simulink library "IOBlock_Library_TTC580"  (R2021a)
settings: Solver=ode45  StartTime=0.0  StopTime=10.0  RelTol=1e-3
PreLoadFcn:
  | addpath(genpath(fileparts(which('IOBlock_Library_TTC580'))));
  | %addpath(genpath(fileparts(which('IOBlock_Library_TTC580.mdl'))))
  | try
  | addpath(genpath([fileparts(which('IOBlock_Library_TTC580')),'\..\DBC_Importer']));
  | addpath(genpath([fileparts(which('IOBlock_Library_TTC580')),'\..\EEPROM_Importer']));
  | addpath(genpath([fileparts(which('IOBlock_Library_TTC580')),'\..\UserDoc']));
  | catch
  | warning('IOBlock_Library_TTC580: add path to DBC_Importer and EEPROM_Importer manually');
  | end
  | try
  | if exist('..\CustomPackage\scripts\OpenAllPackages.m','file')
  |      run('..\CustomPackage\scripts\OpenAllPackages.m'); %always available, ggf. empty
  | end
  | catch
  | warning('A problem occurred opening automatically the CustomPackage. Please open libraries manually');
  | end
  | try
  | set_param(0,'EditorSmartEditingHotParam','off');
  | catch
  | warning('Simlink preferences for ''Edit key parameter when adding new blocks'' needs to be unchecked manually');
  | end
undefined symbols (not defined in the file or in its folder): ADC_Absolute_10V, ADC_Absolute_32V, ADC_Absolute_5V, ADC_BoardTemp, ADC_ChannelInit, ADC_Current, ADC_Get, ADC_K15_, ADC_Ratiometric_10V, ADC_Ratiometric_5V, ADC_Resistive, ADC_SensorSupply, ADC_UBAT, bit_packing, bit_unpacking, CAN_ConfigMsg, compare2error, compare2FET_PROT_REENABLE, crc32_calc_intern, CRC32_EEPROM_Read, CRC32_EEPROM_Write, DIAG_EnterSafestate, DIAG_Status, DIAG_Status_internal, EEPROM_Mirror, EEPROM_Read, EEPROM_Read_OffsetIn, EEPROM_Read_Raw, EEPROM_Write, EEPROM_Write_OffsetIn, EEPROM_Write_Raw, EnterSafestate, FPU_Handler, Get_DI, Get_DI_VarThreshold, Get_K15_, Get_Pulse_Freq_Curr, Get_Pulse_Freq_Volt, Get_WakeUp, GetDateAndTime, IO_ADC_ResetProtection, IO_Blk_Lib_TTC500, IO_CAN_ReadMsg, IO_CAN_WriteMsg, IO_DI_Get, IO_DI_Init, IO_DI_Init_Var, IO_DO_GetCur, IO_DO_GetVoltage, IO_DO_Init, IO_DO_ResetProtection, IO_DO_Set, IO_Driver_GetSerialNumber, IO_Driver_GetVersionOfDriver, IO_Driver_GetVersionOfFPGA, IO_EEPROM_GetStatus, IO_EEPROM_Init, IO_EEPROM_Read_raw, IO_EEPROM_Write, IO_EEPROM_Write_OffsetIn ... (+73)
libraries: simulink x43
(part 2 of 18)

== system IOBlock_Library_TTC580/CAN  Blocks TTC580 IOlib ==
  OR_TX : S-Function  FunctionName=sfix_bitop  Parameters=UseBitMask,NumInputPorts,BitMask,BitMaskRealWorld,logicop  SFunctionDeploymentMode=off  EnableBusSupport=off  mask(Bitwise Operator){logicop=OR, UseBitMask=off, NumInputPorts=2, BitMask=bin2dec('11011001'), BitMaskRealWorld=Stored Integer}
      mask prompts: logicop "Operator:"; UseBitMask "Use bit mask ..."; NumInputPorts "Number of input ports:"; BitMask "Bit Mask"; BitMaskRealWorld "Treat mask as:"
      mask help:
      | Perform the specified bitwise operation on the inputs. The output data type should represent zero exactly.
      | CAN buffer-outputs of the bit_packing blocks may be merged to a single CAN buffer (uint32[2]) which may be sent out by CAN_Write blocks.
      mask init:
      | if UseBitMask
      |   [m,n] = size(BitMask);
      |   if ischar(BitMask)
      |     len = m;
      |     n = 1;
      |   else
      |     len = m * n;
      |   end
      |   internalBitMask = zeros(m,n);
      |   if isnumeric(BitMask)
      |     for i=1:len,
      |       internalBitMask(i) = BitMask(i);
      |     end
      |   elseif ischar(BitMask)
      |     for i=1:m,
      |       internalBitMask(i) = hex2dec(BitMask(i,:));
      |     end
      |   elseif iscell(BitMask)
      |     for i=1:len,
      |       if isnumeric( BitMask{i} )
      |         internalBitMask(i) = BitMask{i};
      |       elseif ischar( BitMask{i} )
      |         internalBitMask(i) = hex2dec(BitMask{i});
      |       else
      |         errordlg(['Data type is not supported at cell item ', num2str(i) ]);
      |       end
      |     end
      |   end
      |   BitMask = internalBitMask;
      |   if len == 1
      |      if BitMaskRealWorld == 1 || BitMask(1) < 0
      |        str=num2str(BitMask(1));
      |      else
      |        str=['0x',dec2hex(floor(BitMask(1)))];
      |      end
      |   else
      |      str='Masks';
      |   end
      | else
      |   BitMask = 0;
      |   str='';
      | end
      mask TypeOptions logicop: AND | OR | NAND | NOR | XOR | NOT
      mask Callback logicop: fixptdialog(gcbh)
      mask Callback UseBitMask: fixptdialog(gcbh)
      mask TypeOptions BitMaskRealWorld: Real World Value | Stored Integer
      mask Display: fprintf(['Bitwise\n',logicop,'\n',str])
  ReadMsg_CAN : Subsystem  LoadFcn=|  mask(ReadMsg_CAN_Code){SampleTime=-1, ttlib=IO_Blk_Lib_TTC500, ttDescription=ReadMsg_CAN, tt_iolib_version=0.26, channel=IO_CAN_CHANNEL_0, mode=IO_CAN_MSG_READ, id_format=IO_CAN_STD_FRAME, id=hex2dec('123')}
      | try
      | %
      | %Upgrade Information - standard BEGIN
      | new_color = 'blue';
      | new_ver = '0.26';
      | act_ver = get_param(gcb,'tt_iolib_version');
      | if not(strcmp(act_ver,new_ver))
      |     disp(['Upgrade block: ',gcb,char(10),'       Version: ',act_ver,' to ',new_ver]);
      |     %switch - case for specific upgrade information e.g. additional parameter required 
      |     %Change appearance and version information
      |     set_param(gcb,'ForegroundColor',new_color);
      |     set_param(gcb,'tt_iolib_version',new_ver);
      | end
      | %Upgrade Information - standard END
      | catch
      | %Standard catch section BEGIN
      | errordlg('An error occurred in a callback of the TTC580-BlockLib. Please open the Diagnostic Viewer for further details');
      | disp(' ');
      | disp('------------------------------------------------------------');
      | disp('An error occurred in a callback of the TTC580-BlockLib.');
      | disp(['Please check the parameters in the mask of ',gcb]);
      | disp('If you do not encounter any violations, then please '); 
      | disp('copy the following lines and report this to support@ttcontrol.com ');
      | disp('<< begin of error message dump >>');
      | disp(['Version of TTC580-BlockLib: ', get_param(gcb,'tt_iolib_version')]);
      | disp(get_param(gcb,'ttDescription'));
      | disp(gcb);
      | x=lasterror;disp(x.message);
      | disp(get_param(gcb,'MaskValues'));
      | disp(version);
      | disp(computer);
      | disp('<< end of error message dump >>');
      | disp('------------------------------------------------------------');
      | disp(' ');
      | %Standard catch section END
      | end
      mask help: Reads a message from a given message object.
      mask init: same as IOBlock_Library_TTC580/ADC Blocks TTC580 IOlib/ADC_Absolute_10V
      settings: CopyFcn=%deleted
      mask Help: web([which('usermanual.html'),'#',lower(get_param(gcb,'ttDescription'))])
      mask TypeOptions channel: IO_CAN_CHANNEL_0  | IO_CAN_CHANNEL_1 | IO_CAN_CHANNEL_2 | IO_CAN_CHANNEL_3 | IO_CAN_CHANNEL_4 | IO_CAN_CHANNEL_5 | IO_CAN_CHANNEL_6
      mask Callback channel: %
      mask Callback mode: %
      mask TypeOptions id_format: IO_CAN_STD_FRAME | IO_CAN_EXT_FRAME
      mask Callback id_format: %
      mask Callback id: %
  ReadMsg_CAN_derated : Subsystem  LoadFcn=|  mask(ReadMsg_CAN_derated_Code){SampleTime=-1, ttlib=IO_Blk_Lib_TTC500, ttDescription=ReadMsg_CAN_derated, tt_iolib_version=0.26, channel=IO_CAN_CHANNEL_0, mode=IO_CAN_MSG_READ, id_format=IO_CAN_STD_FRAME, id=hex2dec('123'), derate=10}
      | try
      | %
      | %Upgrade Information - standard BEGIN
      | new_color = 'blue';
      | new_ver = '0.26';
      | act_ver = get_param(gcb,'tt_iolib_version');
      | if not(strcmp(act_ver,new_ver))
      |     disp(['Upgrade block: ',gcb,char(10),'       Version: ',act_ver,' to ',new_ver]);
      |     %switch - case for specific upgrade information e.g. additional parameter required 
      |     %Change appearance and version information
      |     set_param(gcb,'ForegroundColor',new_color);
      |     set_param(gcb,'tt_iolib_version',new_ver);
      | end
      | %Upgrade Information - standard END
      | catch
      | %Standard catch section BEGIN
      | errordlg('An error occurred in a callback of the TTC580-BlockLib. Please open the Diagnostic Viewer for further details');
      | disp(' ');
      | disp('------------------------------------------------------------');
      | disp('An error occurred in a callback of the TTC580-BlockLib.');
      | disp(['Please check the parameters in the mask of ',gcb]);
      | disp('If you do not encounter any violations, then please '); 
      | disp('copy the following lines and report this to support@ttcontrol.com ');
      | disp('<< begin of error message dump >>');
      | disp(['Version of TTC580-BlockLib: ', get_param(gcb,'tt_iolib_version')]);
      | disp(get_param(gcb,'ttDescription'));
      | disp(gcb);
      | x=lasterror;disp(x.message);
      | disp(get_param(gcb,'MaskValues'));
      | disp(version);
      | disp(computer);
      | disp('<< end of error message dump >>');
      | disp('------------------------------------------------------------');
      | disp(' ');
      | %Standard catch section END
      | end
      mask help:
      | Representation of the ReadMsg_CAN function call, with derate
      | functionality.
      mask init: same as IOBlock_Library_TTC580/ADC Blocks TTC580 IOlib/ADC_Absolute_10V
      settings: CopyFcn=%deleted
      mask Help: web([which('usermanual.html'),'#',lower(get_param(gcb,'ttDescription'))])
      mask TypeOptions channel: IO_CAN_CHANNEL_0  | IO_CAN_CHANNEL_1 | IO_CAN_CHANNEL_2 | IO_CAN_CHANNEL_3 | IO_CAN_CHANNEL_4 | IO_CAN_CHANNEL_5 | IO_CAN_CHANNEL_6
      mask Callback channel: %
      mask Callback mode: %
      mask TypeOptions id_format: IO_CAN_STD_FRAME | IO_CAN_EXT_FRAME
      mask Callback id_format: %
      mask Callback id: %
      mask Callback derate: %
  WriteMsg_CAN : Subsystem  LoadFcn=|  mask(WriteMsg_CAN_Code){SampleTime=-1, ttlib=IO_Blk_Lib_TTC500, ttDescription=WriteMsg_CAN, tt_iolib_version=0.26, channel=IO_CAN_CHANNEL_0, mode=IO_CAN_MSG_WRITE, id_format=IO_CAN_STD_FRAME, id=hex2dec('123'), length=8}
      | try
      | %
      | %Upgrade Information - standard BEGIN
      | new_color = 'blue';
      | new_ver = '0.26';
      | act_ver = get_param(gcb,'tt_iolib_version');
      | if not(strcmp(act_ver,new_ver))
      |     disp(['Upgrade block: ',gcb,char(10),'       Version: ',act_ver,' to ',new_ver]);
      |     %switch - case for specific upgrade information e.g. additional parameter required 
      |     %Change appearance and version information
      |     set_param(gcb,'ForegroundColor',new_color);
      |     set_param(gcb,'tt_iolib_version',new_ver);
      | end
      | %Upgrade Information - standard END
      | catch
      | %Standard catch section BEGIN
      | errordlg('An error occurred in a callback of the TTC580-BlockLib. Please open the Diagnostic Viewer for further details');
      | disp(' ');
      | disp('------------------------------------------------------------');
      | disp('An error occurred in a callback of the TTC580-BlockLib.');
      | disp(['Please check the parameters in the mask of ',gcb]);
      | disp('If you do not encounter any violations, then please '); 
      | disp('copy the following lines and report this to support@ttcontrol.com ');
      | disp('<< begin of error message dump >>');
      | disp(['Version of TTC580-BlockLib: ', get_param(gcb,'tt_iolib_version')]);
      | disp(get_param(gcb,'ttDescription'));
      | disp(gcb);
      | x=lasterror;disp(x.message);
      | disp(get_param(gcb,'MaskValues'));
      | disp(version);
      | disp(computer);
      | disp('<< end of error message dump >>');
      | disp('------------------------------------------------------------');
      | disp(' ');
      | %Standard catch section END
      | end
      mask help: Transmits a CAN message, using the given channel and message object.
      mask init: same as IOBlock_Library_TTC580/ADC Blocks TTC580 IOlib/ADC_Absolute_10V
      settings: CopyFcn=%deleted
      mask Help: web([which('usermanual.html'),'#',lower(get_param(gcb,'ttDescription'))])
      mask TypeOptions channel: IO_CAN_CHANNEL_0  | IO_CAN_CHANNEL_1 | IO_CAN_CHANNEL_2 | IO_CAN_CHANNEL_3 | IO_CAN_CHANNEL_4 | IO_CAN_CHANNEL_5 | IO_CAN_CHANNEL_6
      mask Callback channel: %
      mask Callback mode: %
      mask TypeOptions id_format: IO_CAN_STD_FRAME | IO_CAN_EXT_FRAME
      mask Callback id_format: %
      mask Callback id: %
      mask Callback length: %
  WriteMsg_CAN_derated : Subsystem  LoadFcn=|  mask(WriteMsg_CAN_derated_Code){SampleTime=-1, ttlib=IO_Blk_Lib_TTC500, ttDescription=WriteMsg_CAN_derated, tt_iolib_version=0.26, channel=IO_CAN_CHANNEL_0, mode=IO_CAN_MSG_WRITE, id_format=IO_CAN_STD_FRAME, id=hex2dec('123'), length=8, derate=10}
      | try
      | %
      | %Upgrade Information - standard BEGIN
      | new_color = 'blue';
      | new_ver = '0.26';
      | act_ver = get_param(gcb,'tt_iolib_version');
      | if not(strcmp(act_ver,new_ver))
      |     disp(['Upgrade block: ',gcb,char(10),'       Version: ',act_ver,' to ',new_ver]);
      |     %switch - case for specific upgrade information e.g. additional parameter required 
      |     %Change appearance and version information
      |     set_param(gcb,'ForegroundColor',new_color);
      |     set_param(gcb,'tt_iolib_version',new_ver);
      | end
      | %Upgrade Information - standard END
      | catch
      | %Standard catch section BEGIN
      | errordlg('An error occurred in a callback of the TTC580-BlockLib. Please open the Diagnostic Viewer for further details');
      | disp(' ');
      | disp('------------------------------------------------------------');
      | disp('An error occurred in a callback of the TTC580-BlockLib.');
      | disp(['Please check the parameters in the mask of ',gcb]);
      | disp('If you do not encounter any violations, then please '); 
      | disp('copy the following lines and report this to support@ttcontrol.com ');
      | disp('<< begin of error message dump >>');
      | disp(['Version of TTC580-BlockLib: ', get_param(gcb,'tt_iolib_version')]);
      | disp(get_param(gcb,'ttDescription'));
      | disp(gcb);
      | x=lasterror;disp(x.message);
      | disp(get_param(gcb,'MaskValues'));
      | disp(version);
      | disp(computer);
      | disp('<< end of error message dump >>');
      | disp('------------------------------------------------------------');
      | disp(' ');
      | %Standard catch section END
      | end
      mask help:
      | Representation of the WriteMsg_CAN function call with derate
      | functionality.
      mask init: same as IOBlock_Library_TTC580/ADC Blocks TTC580 IOlib/ADC_Absolute_10V
      settings: CopyFcn=%deleted
      mask Help: web([which('usermanual.html'),'#',lower(get_param(gcb,'ttDescription'))])
      mask TypeOptions channel: IO_CAN_CHANNEL_0  | IO_CAN_CHANNEL_1 | IO_CAN_CHANNEL_2 | IO_CAN_CHANNEL_3 | IO_CAN_CHANNEL_4 | IO_CAN_CHANNEL_5 | IO_CAN_CHANNEL_6
      mask Callback channel: %
      mask Callback mode: %
      mask TypeOptions id_format: IO_CAN_STD_FRAME | IO_CAN_EXT_FRAME
      mask Callback id_format: %
      mask Callback id: %
      mask Callback length: %
      mask Callback derate: %
  bit_packing : Subsystem  LoadFcn=|  mask(bit_packing_Code){SampleTime=-1, ttlib=IO_Blk_Lib_TTC500, ttDescription=bit_packing, tt_iolib_version=0.26, Endianness=little, Format=unsigned, Inversion=off, Startbit=0, Width_bits=8, Factor=1.0, Offset=0.0}
      | try
      | %
      | %Upgrade Information - standard BEGIN
      | new_color = 'blue';
      | new_ver = '0.26';
      | act_ver = get_param(gcb,'tt_iolib_version');
      | if not(strcmp(act_ver,new_ver))
      |     disp(['Upgrade block: ',gcb,char(10),'       Version: ',act_ver,' to ',new_ver]);
      |     %switch - case for specific upgrade information e.g. additional parameter required 
      |     %Change appearance and version information
      |     set_param(gcb,'ForegroundColor',new_color);
      |     set_param(gcb,'tt_iolib_version',new_ver);
      | end
      | %Upgrade Information - standard END
      | catch
      | %Standard catch section BEGIN
      | errordlg('An error occurred in a callback of the TTC580-BlockLib. Please open the Diagnostic Viewer for further details');
      | disp(' ');
      | disp('------------------------------------------------------------');
      | disp('An error occurred in a callback of the TTC580-BlockLib.');
      | disp(['Please check the parameters in the mask of ',gcb]);
      | disp('If you do not encounter any violations, then please '); 
      | disp('copy the following lines and report this to support@ttcontrol.com ');
      | disp('<< begin of error message dump >>');
      | disp(['Version of TTC580-BlockLib: ', get_param(gcb,'tt_iolib_version')]);
      | disp(get_param(gcb,'ttDescription'));
      | disp(gcb);
      | x=lasterror;disp(x.message);
      | disp(get_param(gcb,'MaskValues'));
      | disp(version);
      | disp(computer);
      | disp('<< end of error message dump >>');
      | disp('------------------------------------------------------------');
      | disp(' ');
      | %Standard catch section END
      | end
      mask help:
      | Block to prepare CAN-transmition at specified position within 64bit field.
      | For "Factor" and "Offset" the definition of Vector's CANdb applies:
      | [Physical value] = ( [Raw value] * [Factor] ) + [Offset]
      | with Raw value of a signal being the value as it is transmitted in the CAN-network.
      | Verification capabilities are supported.
      mask init: same as IOBlock_Library_TTC580/ADC Blocks TTC580 IOlib/ADC_Absolute_10V
      settings: CopyFcn=%deleted
      mask Help: web([which('usermanual.html'),'#',lower(get_param(gcb,'ttDescription'))])
      mask TypeOptions Endianness: big | little
      mask Callback Endianness: %
      mask TypeOptions Format: unsigned | signed | real32
      mask Callback Format: %
      mask Callback Inversion: %
      mask Callback Startbit: %
      mask Callback Width_bits: %
      mask Callback Factor: %
      mask Callback Offset: %
  bit_unpacking : Subsystem  LoadFcn=|  mask(bit_unpacking_Code){SampleTime=-1, ttlib=IO_Blk_Lib_TTC500, ttDescription=bit_unpacking, tt_iolib_version=0.26, Endianness=little, Format=unsigned, Inversion=off, Startbit=0, Width_bits=8, Factor=1.0, Offset=0.0}
      | try
      | %
      | %Upgrade Information - standard BEGIN
      | new_color = 'blue';
      | new_ver = '0.26';
      | act_ver = get_param(gcb,'tt_iolib_version');
      | if not(strcmp(act_ver,new_ver))
      |     disp(['Upgrade block: ',gcb,char(10),'       Version: ',act_ver,' to ',new_ver]);
      |     %switch - case for specific upgrade information e.g. additional parameter required 
      |     %Change appearance and version information
      |     set_param(gcb,'ForegroundColor',new_color);
      |     set_param(gcb,'tt_iolib_version',new_ver);
      | end
      | %Upgrade Information - standard END
      | catch
      | %Standard catch section BEGIN
      | errordlg('An error occurred in a callback of the TTC580-BlockLib. Please open the Diagnostic Viewer for further details');
      | disp(' ');
      | disp('------------------------------------------------------------');
      | disp('An error occurred in a callback of the TTC580-BlockLib.');
      | disp(['Please check the parameters in the mask of ',gcb]);
      | disp('If you do not encounter any violations, then please '); 
      | disp('copy the following lines and report this to support@ttcontrol.com ');
      | disp('<< begin of error message dump >>');
      | disp(['Version of TTC580-BlockLib: ', get_param(gcb,'tt_iolib_version')]);
      | disp(get_param(gcb,'ttDescription'));
      | disp(gcb);
      | x=lasterror;disp(x.message);
      | disp(get_param(gcb,'MaskValues'));
      | disp(version);
      | disp(computer);
      | disp('<< end of error message dump >>');
      | disp('------------------------------------------------------------');
      | disp(' ');
      | %Standard catch section END
      | end
      mask help:
      | Block to read in CAN signal from a specified position within 64bit field.
      | For "Factor" and "Offset" the definition of Vector's CANdb applies:
      | [Physical value] = ( [Raw value] * [Factor] ) + [Offset]
      | with Raw value of a signal being the value as it is transmitted in the CAN-network
      | Verification capabilities are supported.
      mask init: same as IOBlock_Library_TTC580/ADC Blocks TTC580 IOlib/ADC_Absolute_10V
      settings: CopyFcn=%deleted
      mask Help: web([which('usermanual.html'),'#',lower(get_param(gcb,'ttDescription'))])
      mask TypeOptions Endianness: big | little
      mask Callback Endianness: %
      mask TypeOptions Format: unsigned | signed | real32
      mask Callback Format: %
      mask Callback Inversion: %
      mask Callback Startbit: %
      mask Callback Width_bits: %
      mask Callback Factor: %
      mask Callback Offset: %

== system IOBlock_Library_TTC580/DIO Blocks TTC580 IOlib ==
  Get_DI : Subsystem  LoadFcn=|  mask(Get_DI_Code){SampleTime=-1, ttlib=IO_Blk_Lib_TTC500, ttDescription=Get_DI, tt_iolib_version=0.26, di_channel=IO_DI_00, pupd=IO_DI_PU_10K}
      | try
      | %
      | %Upgrade Information - standard BEGIN
      | new_color = 'blue';
      | new_ver = '0.26';
      | act_ver = get_param(gcb,'tt_iolib_version');
      | if not(strcmp(act_ver,new_ver))
      |     disp(['Upgrade block: ',gcb,char(10),'       Version: ',act_ver,' to ',new_ver]);
      |     %switch - case for specific upgrade information e.g. additional parameter required 
      |     %Change appearance and version information
      |     set_param(gcb,'ForegroundColor',new_color);
      |     set_param(gcb,'tt_iolib_version',new_ver);
      | end
      | %Upgrade Information - standard END
      | catch
      | %Standard catch section BEGIN
      | errordlg('An error occurred in a callback of the TTC580-BlockLib. Please open the Diagnostic Viewer for further details');
      | disp(' ');
      | disp('------------------------------------------------------------');
      | disp('An error occurred in a callback of the TTC580-BlockLib.');
      | disp(['Please check the parameters in the mask of ',gcb]);
      | disp('If you do not encounter any violations, then please '); 
      | disp('copy the following lines and report this to support@ttcontrol.com ');
      | disp('<< begin of error message dump >>');
      | disp(['Version of TTC580-BlockLib: ', get_param(gcb,'tt_iolib_version')]);
      | disp(get_param(gcb,'ttDescription'));
      | disp(gcb);
      | x=lasterror;disp(x.message);
      | disp(get_param(gcb,'MaskValues'));
      | disp(version);
      | disp(computer);
      | disp('<< end of error message dump >>');
      | disp('------------------------------------------------------------');
      | disp(' ');
      | %Standard catch section END
      | end
      mask help: Gets the value of a digital input
      mask init: same as IOBlock_Library_TTC580/ADC Blocks TTC580 IOlib/ADC_Absolute_10V
      settings: CopyFcn=%deleted
      mask Help: web([which('usermanual.html'),'#',lower(get_param(gcb,'ttDescription'))])
      mask TypeOptions di_channel: IO_DI_00 | IO_DI_01 | IO_DI_02 | IO_DI_03 | IO_DI_04 | IO_DI_05 | IO_DI_06 | IO_DI_07 | IO_DI_08 | IO_DI_09 | IO_DI_10 | IO_DI_11 | IO_DI_12 | IO_DI_13 | IO_DI_14 | IO_DI_15 | IO_DI_16 | IO_DI_17 | IO_DI_18 | IO_DI_19 | IO_DI_20 | IO_DI_21 | IO_DI_22 | IO_DI_23 | IO_DI_24 | IO_DI_25 | IO_DI_26 | IO_DI_27 | IO_DI_28 | IO_DI_29 | IO_DI_30 | IO_DI_31 | IO_DI_32 | IO_DI_33 | IO_DI_34 | IO_DI_35 | IO_DI_36 | IO_DI_37 | IO_DI_38 | IO_DI_39 | IO_DI_40 | IO_DI_41 | IO_DI_42 | IO_DI_43 | IO_DI_44 | IO_DI_45 | IO_DI_46 | IO_DI_47 | IO_DI_48 | IO_DI_49 | IO_DI_50 | IO_DI_51 | IO_DI_52 | IO_DI_53 | IO_DI_54 | IO_DI_55 | IO_DI_56 | IO_DI_57 | IO_DI_58 | IO_DI_59 | IO_DI_60 | IO_DI_61 | IO_DI_62 | IO_DI_63 | IO_DI_64 | IO_DI_65 | IO_DI_66 | IO_DI_67 | IO_DI_68 | IO_DI_69 | IO_DI_70 | IO_DI_71 | IO_DI_72 | IO_DI_73 | IO_DI_74 | IO_DI_75 | IO_DI_76 | IO_DI_77 | IO_DI_78 | IO_DI_79 | IO_DI_80 | IO_DI_81 | IO_DI_82 | IO_DI_83 | IO_DI_84 | IO_DI_85 | IO_DI_86 | IO_DI_87 | IO_DI_88 | IO_DI_89 | IO_DI_90 | IO_DI_91 | IO_DI_92 | IO_DI_93 | IO_DI_94 | IO_DI_95
      mask Callback di_channel:
      | try
      | s_ParameterDecision = 'di_channel'; %Deside on this parameter
      | cc_ValuesDecision={{'IO_DI_00','IO_DI_01','IO_DI_02','IO_DI_03','IO_DI_04','IO_DI_05','IO_DI_06','IO_DI_07','IO_DI_08','IO_DI_09','IO_DI_10','IO_DI_11','IO_DI_12','IO_DI_13','IO_DI_14','IO_DI_15','IO_DI_16','IO_DI_17','IO_DI_18','IO_DI_19','IO_DI_20','IO_DI_21','IO_DI_22','IO_DI_23','IO_DI_24','IO_DI_25','IO_DI_26','IO_DI_27','IO_DI_28','IO_DI_29','IO_DI_30','IO_DI_31','IO_DI_32','IO_DI_33','IO_DI_34','IO_DI_35','IO_DI_48','IO_DI_49','IO_DI_50','IO_DI_51','IO_DI_52','IO_DI_53','IO_DI_54','IO_DI_55','IO_DI_80','IO_DI_81','IO_DI_82','IO_DI_83','IO_DI_84','IO_DI_85','IO_DI_86','IO_DI_87'},
      | {'IO_DI_56','IO_DI_57','IO_DI_58','IO_DI_59','IO_DI_60','IO_DI_61','IO_DI_62','IO_DI_63','IO_DI_64','IO_DI_65','IO_DI_66','IO_DI_67','IO_DI_68','IO_DI_69','IO_DI_70','IO_DI_71'}}; %Positive DescitionValues
      | s_ParameterGrey = 'pupd'; %Gray out this
      | c_ValueGrey = {'IO_DI_PU_10K','IO_DI_PD_10K'};   %Fixed value
      | %trim
      | s_ParameterDecision = strtrim(s_ParameterDecision);
      | cc_ValuesDecision = strtrim(cc_ValuesDecision);
      | s_ParameterGrey = strtrim(s_ParameterGrey);
      | c_ValueGrey = strtrim(c_ValueGrey);
      | c_MaskEnables=get_param(gcb,'MaskEnables');
      | %check consistency
      | if length(cc_ValuesDecision)~= length(c_ValueGrey),disp('DevCode: 012');end
      | idx=strmatch(s_ParameterGrey,get_param(gcb,'MaskNames'));
      | c_MaskEnables{idx}='on'; %default
      |     for i = 1: length(cc_ValuesDecision)
      |         if ~isempty(strmatch(get_param(gcb, s_ParameterDecision), cc_ValuesDecision{i},'exact'))
      |            set_param(gcb, s_ParameterGrey, c_ValueGrey{i});
      |            c_MaskEnables{idx}='off';
      |         end
      |     end
      | set_param(gcb,'MaskEnables',c_MaskEnables);
      | catch
      | %Standard catch section BEGIN
      | errordlg('An error occurred in a callback of the TTC580-BlockLib. Please open the Diagnostic Viewer for further details');
      | disp(' ');
      | disp('------------------------------------------------------------');
      | disp('An error occurred in a callback of the TTC580-BlockLib.');
      | disp(['Please check the parameters in the mask of ',gcb]);
      | disp('If you do not encounter any violations, then please ');
      | disp('copy the following lines and report this to support@ttcontrol.com ');
      | disp('<< begin of error message dump >>');
      | disp(['Version of TTC580-BlockLib: ', get_param(gcb,'tt_iolib_version')]);
      | disp(get_param(gcb,'ttDescription'));
      | disp(gcb);
      | x=lasterror;disp(x.message);
      | disp(get_param(gcb,'MaskValues'));
      | disp(version);
      | disp(computer);
      | disp('<< end of error message dump >>');
      | disp('------------------------------------------------------------');
      | disp(' ');
      | %Standard catch section END
      | end
      mask TypeOptions pupd: IO_DI_PU_10K | IO_DI_PD_10K
      mask Callback pupd: %
  Get_DI_VarThreshold : Subsystem  LoadFcn=|  mask(Get_DI_VarThreshold_Code){SampleTime=-1, ttlib=IO_Blk_Lib_TTC500, ttDescription=Get_DI_VarThreshold, tt_iolib_version=0.26, di_channel=IO_DI_56, pupd=IO_DI_PD_10K, low_thresh1_mV=0, low_thresh2_mV=2500, high_thresh1_mV=2500, high_thresh2_mV=32000}
      | try
      | %
      | %Upgrade Information - standard BEGIN
      | new_color = 'blue';
      | new_ver = '0.26';
      | act_ver = get_param(gcb,'tt_iolib_version');
      | if not(strcmp(act_ver,new_ver))
      |     disp(['Upgrade block: ',gcb,char(10),'       Version: ',act_ver,' to ',new_ver]);
      |     %switch - case for specific upgrade information e.g. additional parameter required 
      |     %Change appearance and version information
      |     set_param(gcb,'ForegroundColor',new_color);
      |     set_param(gcb,'tt_iolib_version',new_ver);
      | end
      | %Upgrade Information - standard END
      | catch
      | %Standard catch section BEGIN
      | errordlg('An error occurred in a callback of the TTC580-BlockLib. Please open the Diagnostic Viewer for further details');
      | disp(' ');
      | disp('------------------------------------------------------------');
      | disp('An error occurred in a callback of the TTC580-BlockLib.');
      | disp(['Please check the parameters in the mask of ',gcb]);
      | disp('If you do not encounter any violations, then please '); 
      | disp('copy the following lines and report this to support@ttcontrol.com ');
      | disp('<< begin of error message dump >>');
      | disp(['Version of TTC580-BlockLib: ', get_param(gcb,'tt_iolib_version')]);
      | disp(get_param(gcb,'ttDescription'));
      | disp(gcb);
      | x=lasterror;disp(x.message);
      | disp(get_param(gcb,'MaskValues'));
      | disp(version);
      | disp(computer);
      | disp('<< end of error message dump >>');
      | disp('------------------------------------------------------------');
      | disp(' ');
      | %Standard catch section END
      | end
      mask help: Gets the value of a digital input with an user definable voltage threshold
      mask init: same as IOBlock_Library_TTC580/ADC Blocks TTC580 IOlib/ADC_Absolute_10V
      settings: CopyFcn=%deleted
      mask Help: web([which('usermanual.html'),'#',lower(get_param(gcb,'ttDescription'))])
      mask TypeOptions di_channel: IO_DI_56 | IO_DI_57 | IO_DI_58 | IO_DI_59 | IO_DI_60 | IO_DI_61 | IO_DI_62 | IO_DI_63 | IO_DI_64 | IO_DI_65 | IO_DI_66 | IO_DI_67 | IO_DI_68 | IO_DI_69 | IO_DI_70 | IO_DI_71 | IO_DI_72 | IO_DI_73 | IO_DI_74 | IO_DI_75 | IO_DI_76 | IO_DI_77 | IO_DI_78 | IO_DI_79 | IO_DI_80 | IO_DI_81 | IO_DI_82 | IO_DI_83 | IO_DI_84 | IO_DI_85 | IO_DI_86 | IO_DI_87 | IO_DI_88 | IO_DI_89 | IO_DI_90 | IO_DI_91 | IO_DI_92 | IO_DI_93 | IO_DI_94 | IO_DI_95
      mask Callback di_channel:
      | try
      | s_ParameterDecision = 'di_channel'; %Deside on this parameter
      | cc_ValuesDecision={{'IO_DI_00','IO_DI_01','IO_DI_02','IO_DI_03','IO_DI_04','IO_DI_05','IO_DI_06','IO_DI_07','IO_DI_08','IO_DI_09','IO_DI_10','IO_DI_11','IO_DI_12','IO_DI_13','IO_DI_14','IO_DI_15','IO_DI_16','IO_DI_17','IO_DI_18','IO_DI_19','IO_DI_20','IO_DI_21','IO_DI_22','IO_DI_23','IO_DI_24','IO_DI_25','IO_DI_26','IO_DI_27','IO_DI_28','IO_DI_29','IO_DI_30','IO_DI_31','IO_DI_32','IO_DI_33','IO_DI_34','IO_DI_35','IO_DI_48','IO_DI_49','IO_DI_50','IO_DI_51','IO_DI_52','IO_DI_53','IO_DI_54','IO_DI_55','IO_DI_80','IO_DI_81','IO_DI_82','IO_DI_83','IO_DI_84','IO_DI_85','IO_DI_86','IO_DI_87'},
      | {'IO_DI_56','IO_DI_57','IO_DI_58','IO_DI_59','IO_DI_60','IO_DI_61','IO_DI_62','IO_DI_63','IO_DI_64','IO_DI_65','IO_DI_66','IO_DI_67','IO_DI_68','IO_DI_69','IO_DI_70','IO_DI_71'}}; %Positive DescitionValues
      | s_ParameterGrey = 'pupd'; %Gray out this
      | c_ValueGrey = {'IO_DI_PU_10K','IO_DI_PD_10K'};   %Fixed value
      | %trim
      | s_ParameterDecision = strtrim(s_ParameterDecision);
      | cc_ValuesDecision = strtrim(cc_ValuesDecision);
      | s_ParameterGrey = strtrim(s_ParameterGrey);
      | c_ValueGrey = strtrim(c_ValueGrey);
      | c_MaskEnables=get_param(gcb,'MaskEnables');
      | %check consistency
      | if length(cc_ValuesDecision)~= length(c_ValueGrey),disp('DevCode: 012');end
      | idx=strmatch(s_ParameterGrey,get_param(gcb,'MaskNames'));
      | c_MaskEnables{idx}='on'; %default
      |     for i = 1: length(cc_ValuesDecision)
      |         if ~isempty(strmatch(get_param(gcb, s_ParameterDecision), cc_ValuesDecision{i},'exact'))
      |            set_param(gcb, s_ParameterGrey, c_ValueGrey{i});
      |            c_MaskEnables{idx}='off';
      |         end
      |     end
      | set_param(gcb,'MaskEnables',c_MaskEnables);
      | catch
      | %Standard catch section BEGIN
      | errordlg('An error occurred in a callback of the TTC580-BlockLib. Please open the Diagnostic Viewer for further details');
      | disp(' ');
      | disp('------------------------------------------------------------');
      | disp('An error occurred in a callback of the TTC580-BlockLib.');
      | disp(['Please check the parameters in the mask of ',gcb]);
      | disp('If you do not encounter any violations, then please ');
      | disp('copy the following lines and report this to support@ttcontrol.com ');
      | disp('<< begin of error message dump >>');
      | disp(['Version of TTC580-BlockLib: ', get_param(gcb,'tt_iolib_version')]);
      | disp(get_param(gcb,'ttDescription'));
      | disp(gcb);
      | x=lasterror;disp(x.message);
      | disp(get_param(gcb,'MaskValues'));
      | disp(version);
      | disp(computer);
      | disp('<< end of error message dump >>');
      | disp('------------------------------------------------------------');
      | disp(' ');
      | %Standard catch section END
      | end
      mask TypeOptions pupd: IO_DI_PU_10K | IO_DI_PD_10K
      mask Callback pupd: %
      mask Callback low_thresh1_mV: %
      mask Callback low_thresh2_mV: %
      mask Callback high_thresh1_mV: %
      mask Callback high_thresh2_mV: %
  Get_K15_ : Subsystem  LoadFcn=|  mask(Get_K15__Code){SampleTime=-1, ttlib=IO_Blk_Lib_TTC500, ttDescription=Get_K15_, tt_iolib_version=0.26, pin=IO_K15}
      | try
      | %
      | %Upgrade Information - standard BEGIN
      | new_color = 'blue';
      | new_ver = '0.26';
      | act_ver = get_param(gcb,'tt_iolib_version');
      | if not(strcmp(act_ver,new_ver))
      |     disp(['Upgrade block: ',gcb,char(10),'       Version: ',act_ver,' to ',new_ver]);
      |     %switch - case for specific upgrade information e.g. additional parameter required 
      |     %Change appearance and version information
      |     set_param(gcb,'ForegroundColor',new_color);
      |     set_param(gcb,'tt_iolib_version',new_ver);
      | end
      | %Upgrade Information - standard END
      | catch
      | %Standard catch section BEGIN
      | errordlg('An error occurred in a callback of the TTC580-BlockLib. Please open the Diagnostic Viewer for further details');
      | disp(' ');
      | disp('------------------------------------------------------------');
      | disp('An error occurred in a callback of the TTC580-BlockLib.');
      | disp(['Please check the parameters in the mask of ',gcb]);
      | disp('If you do not encounter any violations, then please '); 
      | disp('copy the following lines and report this to support@ttcontrol.com ');
      | disp('<< begin of error message dump >>');
      | disp(['Version of TTC580-BlockLib: ', get_param(gcb,'tt_iolib_version')]);
      | disp(get_param(gcb,'ttDescription'));
      | disp(gcb);
      | x=lasterror;disp(x.message);
      | disp(get_param(gcb,'MaskValues'));
      | disp(version);
      | disp(computer);
      | disp('<< end of error message dump >>');
      | disp('------------------------------------------------------------');
      | disp(' ');
      | %Standard catch section END
      | end
      mask help: Returns the state of K15: OFF (=0) or ON(=1)
      mask init: same as IOBlock_Library_TTC580/ADC Blocks TTC580 IOlib/ADC_Absolute_10V
      settings: CopyFcn=%deleted
      mask Help: web([which('usermanual.html'),'#',lower(get_param(gcb,'ttDescription'))])
      mask Callback pin: %
  Get_WakeUp : Subsystem  LoadFcn=|  mask(Get_WakeUp_Code){SampleTime=-1, ttlib=IO_Blk_Lib_TTC500, ttDescription=Get_WakeUp, tt_iolib_version=0.26, pin=IO_WAKEUP}
      | try
      | %
      | %Upgrade Information - standard BEGIN
      | new_color = 'blue';
      | new_ver = '0.26';
      | act_ver = get_param(gcb,'tt_iolib_version');
      | if not(strcmp(act_ver,new_ver))
      |     disp(['Upgrade block: ',gcb,char(10),'       Version: ',act_ver,' to ',new_ver]);
      |     %switch - case for specific upgrade information e.g. additional parameter required 
      |     %Change appearance and version information
      |     set_param(gcb,'ForegroundColor',new_color);
      |     set_param(gcb,'tt_iolib_version',new_ver);
      | end
      | %Upgrade Information - standard END
      | catch
      | %Standard catch section BEGIN
      | errordlg('An error occurred in a callback of the TTC580-BlockLib. Please open the Diagnostic Viewer for further details');
      | disp(' ');
      | disp('------------------------------------------------------------');
      | disp('An error occurred in a callback of the TTC580-BlockLib.');
      | disp(['Please check the parameters in the mask of ',gcb]);
      | disp('If you do not encounter any violations, then please '); 
      | disp('copy the following lines and report this to support@ttcontrol.com ');
      | disp('<< begin of error message dump >>');
      | disp(['Version of TTC580-BlockLib: ', get_param(gcb,'tt_iolib_version')]);
      | disp(get_param(gcb,'ttDescription'));
      | disp(gcb);
      | x=lasterror;disp(x.message);
      | disp(get_param(gcb,'MaskValues'));
      | disp(version);
      | disp(computer);
      | disp('<< end of error message dump >>');
      | disp('------------------------------------------------------------');
      | disp(' ');
      | %Standard catch section END
      | end
      mask help: Returns the state of WakeUp: OFF (=0) or ON(=1)
      mask init: same as IOBlock_Library_TTC580/ADC Blocks TTC580 IOlib/ADC_Absolute_10V
      settings: CopyFcn=%deleted
      mask Help: web([which('usermanual.html'),'#',lower(get_param(gcb,'ttDescription'))])
      mask Callback pin: %
  Set_DO_HighSide : Subsystem  LoadFcn=|  mask(Set_DO_HighSide_Code){SampleTime=-1, ttlib=IO_Blk_Lib_TTC500, ttDescription=Set_DO_HighSide, tt_iolib_version=0.26, do_channel=IO_DO_00, diagnostic=off}
      | try
      | %
      | %Upgrade Information - standard BEGIN
      | new_color = 'blue';
      | new_ver = '0.26';
      | act_ver = get_param(gcb,'tt_iolib_version');
      | if not(strcmp(act_ver,new_ver))
      |     disp(['Upgrade block: ',gcb,char(10),'       Version: ',act_ver,' to ',new_ver]);
      |     %switch - case for specific upgrade information e.g. additional parameter required 
      |     %Change appearance and version information
      |     set_param(gcb,'ForegroundColor',new_color);
      |     set_param(gcb,'tt_iolib_version',new_ver);
      | end
      | %Upgrade Information - standard END
      | catch
      | %Standard catch section BEGIN
      | errordlg('An error occurred in a callback of the TTC580-BlockLib. Please open the Diagnostic Viewer for further details');
      | disp(' ');
      | disp('------------------------------------------------------------');
      | disp('An error occurred in a callback of the TTC580-BlockLib.');
      | disp(['Please check the parameters in the mask of ',gcb]);
      | disp('If you do not encounter any violations, then please '); 
      | disp('copy the following lines and report this to support@ttcontrol.com ');
      | disp('<< begin of error message dump >>');
      | disp(['Version of TTC580-BlockLib: ', get_param(gcb,'tt_iolib_version')]);
      | disp(get_param(gcb,'ttDescription'));
      | disp(gcb);
      | x=lasterror;disp(x.message);
      | disp(get_param(gcb,'MaskValues'));
      | disp(version);
      | disp(computer);
      | disp('<< end of error message dump >>');
      | disp('------------------------------------------------------------');
      | disp(' ');
      | %Standard catch section END
      | end
      mask help: Sets the value of a digital output
      mask init: same as IOBlock_Library_TTC580/ADC Blocks TTC580 IOlib/ADC_Absolute_10V
      settings: CopyFcn=%deleted
      mask Help: web([which('usermanual.html'),'#',lower(get_param(gcb,'ttDescription'))])
      mask TypeOptions do_channel: IO_DO_00 | IO_DO_01 | IO_DO_02 | IO_DO_03 | IO_DO_04 | IO_DO_05 | IO_DO_06 | IO_DO_07 | IO_DO_16 | IO_DO_17 | IO_DO_18 | IO_DO_19 | IO_DO_20 | IO_DO_21 | IO_DO_22 | IO_DO_23 | IO_DO_24 | IO_DO_25 | IO_DO_26 | IO_DO_27 | IO_DO_28 | IO_DO_29 | IO_DO_30 | IO_DO_31 | IO_DO_32 | IO_DO_33 | IO_DO_34 | IO_DO_35 | IO_DO_36 | IO_DO_37 | IO_DO_38 | IO_DO_39 | IO_DO_40 | IO_DO_41 | IO_DO_42 | IO_DO_43 | IO_DO_44 | IO_DO_45 | IO_DO_46 | IO_DO_47 | IO_DO_48 | IO_DO_49 | IO_DO_50 | IO_DO_51 | IO_DO_52 | IO_DO_53 | IO_DO_54 | IO_DO_55 | IO_DO_56 | IO_DO_57 | IO_DO_58 | IO_DO_59
      mask Callback do_channel:
      | try
      | s_ParameterDecision = 'do_channel'; %Deside on this parameter
      | cc_ValuesDecision={{'IO_DO_16','IO_DO_17','IO_DO_18','IO_DO_19','IO_DO_20','IO_DO_21','IO_DO_22','IO_DO_23','IO_DO_24','IO_DO_25','IO_DO_26','IO_DO_27','IO_DO_28','IO_DO_29','IO_DO_30','IO_DO_31','IO_DO_32','IO_DO_33','IO_DO_34','IO_DO_35','IO_DO_36','IO_DO_37','IO_DO_38','IO_DO_39','IO_DO_40','IO_DO_41','IO_DO_42','IO_DO_43','IO_DO_44','IO_DO_45','IO_DO_46','IO_DO_47','IO_DO_48','IO_DO_49','IO_DO_50','IO_DO_51'}}; %Positive DescitionValues
      | s_ParameterGrey = 'diagnostic'; %Gray out this
      | c_ValueGrey = {'off'};   %Fixed value
      | %trim
      | s_ParameterDecision = strtrim(s_ParameterDecision);
      | cc_ValuesDecision = strtrim(cc_ValuesDecision);
      | s_ParameterGrey = strtrim(s_ParameterGrey);
      | c_ValueGrey = strtrim(c_ValueGrey);
      | c_MaskEnables=get_param(gcb,'MaskEnables');
      | %check consistency
      | if length(cc_ValuesDecision)~= length(c_ValueGrey),disp('DevCode: 012');end
      | idx=strmatch(s_ParameterGrey,get_param(gcb,'MaskNames'));
      | c_MaskEnables{idx}='on'; %default
      |     for i = 1: length(cc_ValuesDecision)
      |         if ~isempty(strmatch(get_param(gcb, s_ParameterDecision), cc_ValuesDecision{i},'exact'))
      |            set_param(gcb, s_ParameterGrey, c_ValueGrey{i});
      |            c_MaskEnables{idx}='off';
      |         end
      |     end
      | set_param(gcb,'MaskEnables',c_MaskEnables);
      | catch
      | %Standard catch section BEGIN
      | errordlg('An error occurred in a callback of the TTC580-BlockLib. Please open the Diagnostic Viewer for further details');
      | disp(' ');
      | disp('------------------------------------------------------------');
      | disp('An error occurred in a callback of the TTC580-BlockLib.');
      | disp(['Please check the parameters in the mask of ',gcb]);
      | disp('If you do not encounter any violations, then please ');
      | disp('copy the following lines and report this to support@ttcontrol.com ');
      | disp('<< begin of error message dump >>');
      | disp(['Version of TTC580-BlockLib: ', get_param(gcb,'tt_iolib_version')]);
      | disp(get_param(gcb,'ttDescription'));
      | disp(gcb);
      | x=lasterror;disp(x.message);
      | disp(get_param(gcb,'MaskValues'));
      | disp(version);
      | disp(computer);
      | disp('<< end of error message dump >>');
      | disp('------------------------------------------------------------');
      | disp(' ');
      | %Standard catch section END
      | end
      mask Callback diagnostic: %
  Set_DO_HighSide_Fullfb : Subsystem  LoadFcn=|  mask(Set_DO_HighSide_Fullfb_Code){SampleTime=-1, ttlib=IO_Blk_Lib_TTC500, ttDescription=Set_DO_HighSide_Fullfb, tt_iolib_version=0.26, do_channel=IO_DO_00, diagnostic=off}
      | try
      | %
      | %Upgrade Information - standard BEGIN
      | new_color = 'blue';
      | new_ver = '0.26';
      | act_ver = get_param(gcb,'tt_iolib_version');
      | if not(strcmp(act_ver,new_ver))
      |     disp(['Upgrade block: ',gcb,char(10),'       Version: ',act_ver,' to ',new_ver]);
      |     %switch - case for specific upgrade information e.g. additional parameter required 
      |     %Change appearance and version information
      |     set_param(gcb,'ForegroundColor',new_color);
      |     set_param(gcb,'tt_iolib_version',new_ver);
      | end
      | %Upgrade Information - standard END
      | catch
      | %Standard catch section BEGIN
      | errordlg('An error occurred in a callback of the TTC580-BlockLib. Please open the Diagnostic Viewer for further details');
      | disp(' ');
      | disp('------------------------------------------------------------');
      | disp('An error occurred in a callback of the TTC580-BlockLib.');
      | disp(['Please check the parameters in the mask of ',gcb]);
      | disp('If you do not encounter any violations, then please '); 
      | disp('copy the following lines and report this to support@ttcontrol.com ');
      | disp('<< begin of error message dump >>');
      | disp(['Version of TTC580-BlockLib: ', get_param(gcb,'tt_iolib_version')]);
      | disp(get_param(gcb,'ttDescription'));
      | disp(gcb);
      | x=lasterror;disp(x.message);
      | disp(get_param(gcb,'MaskValues'));
      | disp(version);
      | disp(computer);
      | disp('<< end of error message dump >>');
      | disp('------------------------------------------------------------');
      | disp(' ');
      | %Standard catch section END
      | end
      mask help: Sets the value of a digital output
      mask init: same as IOBlock_Library_TTC580/ADC Blocks TTC580 IOlib/ADC_Absolute_10V
      settings: CopyFcn=%deleted
      mask Help: web([which('usermanual.html'),'#',lower(get_param(gcb,'ttDescription'))])
      mask TypeOptions do_channel: IO_DO_00 | IO_DO_01 | IO_DO_02 | IO_DO_03 | IO_DO_04 | IO_DO_05 | IO_DO_06 | IO_DO_07 | IO_DO_52 | IO_DO_53 | IO_DO_54 | IO_DO_55 | IO_DO_56 | IO_DO_57 | IO_DO_58 | IO_DO_59
      mask Callback do_channel: %
      mask Callback diagnostic: %
  Set_DO_LowSide : Subsystem  LoadFcn=|  mask(Set_DO_LowSide_Code){SampleTime=-1, ttlib=IO_Blk_Lib_TTC500, ttDescription=Set_DO_LowSide, tt_iolib_version=0.26, do_channel=IO_DO_08, diagnostic=off}
      | try
      | %
      | %Upgrade Information - standard BEGIN
      | new_color = 'blue';
      | new_ver = '0.26';
      | act_ver = get_param(gcb,'tt_iolib_version');
      | if not(strcmp(act_ver,new_ver))
      |     disp(['Upgrade block: ',gcb,char(10),'       Version: ',act_ver,' to ',new_ver]);
      |     %switch - case for specific upgrade information e.g. additional parameter required 
      |     %Change appearance and version information
      |     set_param(gcb,'ForegroundColor',new_color);
      |     set_param(gcb,'tt_iolib_version',new_ver);
      | end
      | %Upgrade Information - standard END
      | catch
      | %Standard catch section BEGIN
      | errordlg('An error occurred in a callback of the TTC580-BlockLib. Please open the Diagnostic Viewer for further details');
      | disp(' ');
      | disp('------------------------------------------------------------');
      | disp('An error occurred in a callback of the TTC580-BlockLib.');
      | disp(['Please check the parameters in the mask of ',gcb]);
      | disp('If you do not encounter any violations, then please '); 
      | disp('copy the following lines and report this to support@ttcontrol.com ');
      | disp('<< begin of error message dump >>');
      | disp(['Version of TTC580-BlockLib: ', get_param(gcb,'tt_iolib_version')]);
      | disp(get_param(gcb,'ttDescription'));
      | disp(gcb);
      | x=lasterror;disp(x.message);
      | disp(get_param(gcb,'MaskValues'));
      | disp(version);
      | disp(computer);
      | disp('<< end of error message dump >>');
      | disp('------------------------------------------------------------');
      | disp(' ');
      | %Standard catch section END
      | end
      mask help: Sets the value of a digital output
      mask init: same as IOBlock_Library_TTC580/ADC Blocks TTC580 IOlib/ADC_Absolute_10V
      settings: CopyFcn=%deleted
      mask Help: web([which('usermanual.html'),'#',lower(get_param(gcb,'ttDescription'))])
      mask TypeOptions do_channel: IO_DO_08 | IO_DO_09 | IO_DO_10 | IO_DO_11 | IO_DO_12 | IO_DO_13 | IO_DO_14 | IO_DO_15
      mask Callback do_channel: %
      mask Callback diagnostic: %
